simulink model "four_machine"  (R2020a)
settings: Solver=ode15s  StartTime=0.0  StopTime=20  MaxStep=1/60  RelTol=1e-3  EnableMultiTasking=on
values from neighbouring files (symbols this model uses):
  case_n = i-1    [main_simulations.m]
  d11_step = load_step_size    (= 350)    [main_simulations.m]
  d5_step = 0    [main_simulations.m]
  H = [6.5 6.5 6.175 6.175]*.75    [main_simulations.m]
  kpss = 0.2    [main_simulations.m]
  Tdelay = 0.2    [main_simulations.m]
undefined symbols (not defined in the file or in its folder): D1, d_rad, Delta, K
libraries: powerlib x49, sps_avr x4, powerlib_meascontrol x4, simulink x2, dspsigops x2
(part 1 of 2)
Description:
  | Copyright 2008-2018 The MathWorks, Inc.
settings Model: FPTRunName=Active  ExtModeTrigMode=oneshot  ExtModeArmWhenConnect=off  ExtModeAutoUpdateStatusClock=off  Creator=MathWorks  LastModifiedBy=joakbj
settings DataIOCC: SaveFormat=Array  SaveOutput=off  SaveTime=off  ReturnWorkspaceOutputs=off  TimeSaveName=t  SignalLoggingName=sigsOut
settings OptimizationCC: BlockReduction=off  BooleanDataType=off  ExpressionDepthLimit=2147483647  InitFltsAndDblsToZero=on  LifeSpan=inf
settings DebuggingCC: UnderspecifiedInitializationDetection=Classic  MergeDetectMultiDrivingBlocksExec=none  SignalResolutionControl=TryResolveAllWithWarning  MultiTaskDSMMsg=warning  MultiTaskCondExecSysMsg=none  FcnCallInpInsideContextMsg=warning  UnconnectedInputMsg=none  UnconnectedOutputMsg=none  UnconnectedLineMsg=none  StateNameClashWarn=warning  SFUnexpectedBacktrackingDiag=warning  SFNoUnconditionalDefaultTransitionDiag=warning  SFExecutionAtInitializationDiag=none  ArithmeticOperatorsInVariantConditions=warning
settings HardwareCC: ProdBitPerPointer=32  ProdBitPerSizeT=32  ProdBitPerPtrDiffT=32  ProdLargestAtomicFloat=None  ProdIntDivRoundTo=Undefined  ProdEndianess=Unspecified  ProdWordSize=32  ProdHWDeviceType=32-bit Generic  TargetUnknown=on
settings ModelReferenceCC: PropagateSignalLabelsOutOfModel=off
settings SFSimCC: SimUseLocalCustomCode=off  CustomCodeUndefinedFunction=UseInterfaceOnly
settings RTWCC: RTWUseLocalCustomCode=off
settings CodeAppCC: StateflowObjectComments=on
settings GRTTargetCC: TargetLangStandard=C89/C90 (ANSI)  CombineOutputUpdateFcns=off  GRTInterface=on
settings ConfigComp: CovMetricSettings=dw  CovHtmlReporting=on  CovSaveCumulativeToWorkspaceVar=on  CovSaveSingleToWorkspaceVar=on  CovExternalEMLEnable=off  CovSFcnEnable=off
settings SimscapeCC: SimscapeNormalizeSystem=off

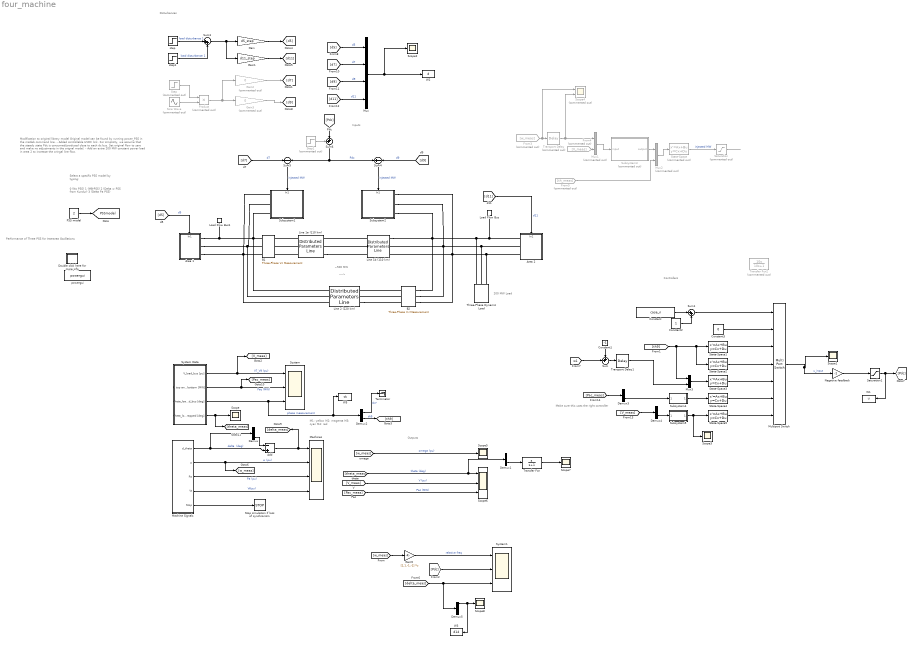
== system four_machine ==
  note: Modification to original library model
      | Original model can be found by running power_PSS in the matlab command line.
      |
      | - Added controllable HVDC link. For simplisity, we assume that the steady state Pdc is
      | consumed/produced close to each dc bus.
      | Set original flow to zero and make no adjustments in the orignal model.
      |
      | - Add an extra 200 MW constant power load in area 2 to increase the oringal line flow.
  note: Make sure this uses the right controller
  note: 200 MW Load
  note: Disturbances
  note: Performance of Three PSS for Interarea Oscillations
  note: M1: yellow
      | M2: magenta
      | M3: cyan
      | M4: red
  note: ---->
  note: ~500 MW
  note: Select a specific PSS model
      | by typing:
  note: 0  (No PSS)
      | 1  (MB-PSS)
      | 2  (Delta w PSS from Kundur)
      | 3  (Delta Pa PSS)
  note: Outputs
  note: Inputs
  note: Controllers
  Add : Sum  Inputs=-+
  Area 1 : Subsystem
      settings: PortSchema="{\"entries\":[{\"content\":{\"sides\":[{\"content\":{\"connectorIds\":[]},\"type\":\"ConnectorPlacement.EquallySpacedRectSide\",\"uuid\":\"61530743-916b-41d3-ae4c-b0f59ade86dc\"},{\"content\":{\"connectorIds\":[\"RConn1\",\"RConn2\",\"RConn3\"],\"side\":\"RIGHT\"},\"type\":\"ConnectorPlacement.EquallySpacedRectSide\",\"uuid\":\"d4cdbb0d-3031-41c4-8349-05093edd83c9\"},{\"content\":{\"connectorIds\":[\"In1\"],\"side\":\"TOP\"},\"type\":\"ConnectorPlacement.EquallySpacedRectSide\",\"uuid\":\"5f7b4922-b9b9-47cc-81cb-58a7e8a20879\"}]},\"type\":\"ConnectorPlacement.EquallySpacedConnector\",\"uuid\":\"5acf2a3c-d6e4-438f-a169-9a860cbc2f6d\"}],\"packageUris\":[\"http://schema.mathworks.com/mf0/Connector/19700101\"],\"version\":\"1.0\"}"
  Area 2 : Subsystem
      settings: PortSchema="{\"entries\":[{\"content\":{\"sides\":[{\"content\":{\"connectorIds\":[\"LConn1\",\"LConn2\",\"LConn3\"]},\"type\":\"ConnectorPlacement.EquallySpacedRectSide\",\"uuid\":\"e7faa0ec-56a1-4760-94c0-742828807d5f\"},{\"content\":{\"connectorIds\":[],\"side\":\"RIGHT\"},\"type\":\"ConnectorPlacement.EquallySpacedRectSide\",\"uuid\":\"ccb950ba-2df4-4215-8f92-1b8fc73c9261\"},{\"content\":{\"connectorIds\":[\"In1\"],\"side\":\"TOP\"},\"type\":\"ConnectorPlacement.EquallySpacedRectSide\",\"uuid\":\"43b0d608-fcb4-47fa-8870-be4e09a9c317\"}]},\"type\":\"ConnectorPlacement.EquallySpacedConnector\",\"uuid\":\"da59aa7b-0e3d-4680-8192-ce0c0266e238\"}],\"packageUris\":[\"http://schema.mathworks.com/mf0/Connector/19700101\"],\"version\":\"1.0\"}"
  B1 : powerlib/Measurements/Three-Phase V-I Measurement  VoltageMeasurement=phase-to-ground  SetLabelV=on  LabelV=Vabc_B1  Vpu=off  VpuLL=off  CurrentMeasurement=yes  SetLabelI=on  LabelI=Iabc_B1  Ipu=off  Pbase=100e6  Vbase=500e3  OutputType=Complex  PhasorSimulation=on  PSBequivalent=0
  B2 : powerlib/Measurements/Three-Phase V-I Measurement  VoltageMeasurement=phase-to-ground  SetLabelV=on  LabelV=Vabc_B2  Vpu=off  VpuLL=off  CurrentMeasurement=yes  SetLabelI=on  LabelI=Iabc_B2  Ipu=off  Pbase=100e6  Vbase=500e3  OutputType=Complex  PhasorSimulation=on  PSBequivalent=0
  Constant : Constant  Value=case_n
  Constant1 : Constant  Value=-1
  Constant2 : Constant
  Constant3 : Constant  Value=0
  Demux : Demux
  Demux{1..4} (4 alike) : Demux  Outputs=2
  Demux5 : Demux
  Double click here for more info : Subsystem
      settings: OpenFcn=showdemo(bdroot(gcb))
      mask Display: disp('?')
  From3 : From  Commented=on  GotoTag=w_meas
  From4 : From  Commented=on  GotoTag=V_meas
  From5 : From  Commented=on  GotoTag=th_meas
  Gain : Gain  Gain=d5_step
  Gain1 : Gain  Gain=d11_step
  Gain2 : Gain  Commented=on  Gain=0
  Gain3 : Gain  Commented=on  Gain=0
  Gain5 : Gain  Gain=[1,1,-1,-1]  Multiplication=Matrix(K*u)
  Line 1a (110 km) : powerlib/Elements/Distributed Parameters Line  Phases=3  Frequency=60  Resistance=[0.0001*529 1.61]  Inductance=[0.001*529/(377) 0.0061]  Capacitance=[0.00175/529/(377) 5.2489e-9]  Length=110  x1=[1.06729153263772e-08 221955.058861017 221954.627346652;376.991118430775 376.991118430775 376.991118430775;1.05676853901888 0.612824326191211 -0.957969932782551]  x2=[8.0985690030452e-09 213828.873062733 213828.517746943;376.991118430775 376.991118430775 376.991118430775;2.81156380356507 0.285316090081509 -1.28547863099569]  x3=[4.33186807668859e-11 672.907969274506 672.908308948858;376.991118430775 376.991118430775 376.991118430775;2.44599649138148 -2.79060184246198 1.92179081798774]  x4=[3.70403487092246e-11 1739.09783381054 1739.09622903984;376.991118430775 376.991118430775 376.991118430775;-0.503630789857306 0.368243197878753 -1.20255060629328]  x5=0.000622431770558027  V1=ones(3,3)  V2=ones(3,3)  I1=ones(3,3)  I2=ones(3,3)  nHarmo=1  Measurements=None
      settings: AttributesFormatString=\n
  Line 1b (110 km) : powerlib/Elements/Distributed Parameters Line  Phases=3  Frequency=60  Resistance=[0.0001*529 1.61]  Inductance=[0.001*529/(377) 0.0061]  Capacitance=[0.00175/529/(377) 5.2489e-9]  Length=110  x1=[8.0985690030452e-09 213828.873062733 213828.517746943;376.991118430775 376.991118430775 376.991118430775;2.81156380356507 0.285316090081509 -1.28547863099569]  x2=[2.03288713597303e-08 224486.996647561 224486.735562946;376.991118430775 376.991118430775 376.991118430775;-2.93072446072062 -0.036243603410852 -1.60703851965793]  x3=[4.90350656664839e-11 690.468793518143 690.469123207699;376.991118430775 376.991118430775 376.991118430775;2.69719045221346 -2.64610173593933 2.06629090472881]  x4=[2.93087705700001e-11 1721.59813744144 1721.59654310193;376.991118430775 376.991118430775 376.991118430775;-0.775070749600102 0.222153439297898 -1.34864036891686]  x5=0.000622431770558027  V1=ones(3,3)  V2=ones(3,3)  I1=ones(3,3)  I2=ones(3,3)  nHarmo=1  Measurements=None
      settings: AttributesFormatString=\n
  Line 2 (220 km) : powerlib/Elements/Distributed Parameters Line  Phases=3  Frequency=60  Resistance=[0.0001*529 1.61]  Inductance=[0.001*529/(377) 0.0061]  Capacitance=[0.00175/529/(377) 5.2489e-9]  Length=220  x1=[1.06729153263771e-08 221955.058861017 221954.627346652;376.991118430775 376.991118430775 376.991118430775;0.822117289689359 0.467311432234616 -1.10348282673915]  x2=[2.03288713597303e-08 224486.996647561 224486.735562946;376.991118430775 376.991118430775 376.991118430775;3.11780959712945 -0.181756497367447 -1.75255141361452]  x3=[3.92860528810386e-11 669.98397742558 669.984311456636;376.991118430775 376.991118430775 376.991118430775;2.21193561854868 -2.93582336415306 1.77656929025843]  x4=[2.78977153806267e-11 1707.24475294082 1707.24317306548;376.991118430775 376.991118430775 376.991118430775;-0.986304993466549 0.0767584445474056 -1.49403536252848]  x5=0.00124486354111605  V1=ones(3,3)  V2=ones(3,3)  I1=ones(3,3)  I2=ones(3,3)  nHarmo=1  Measurements=None
      settings: AttributesFormatString=\n
  Load Flow Bus : powerlib/Measurements/Load Flow Bus  LConnTagsString=a  Phases=single  Connectors=on one side  ID=B2  Vbase=230e3  Vref=1  Vangle=0  VLF=0.976  VLFb=1  VLFc=1  angleLF=-23.74  angleLFb=0  angleLFc=0
      settings: AttributesFormatString=%<ID>\n%<Vbase>V\n%<VLF>pu\n%<angleLF>deg.
  Load Flow Bus1 : powerlib/Measurements/Load Flow Bus  LConnTagsString=a  Phases=single  Connectors=on one side  ID=B1  Vbase=230e3  Vref=1  Vangle=0  VLF=0.965  VLFb=1  VLFc=1  angleLF=13.45  angleLFb=0  angleLFc=0
      settings: AttributesFormatString=%<ID>\n%<Vbase>V\n%<VLF>pu\n%<angleLF>deg.
  Machine Signals : Subsystem
  Machines : Scope  NumInputPorts=4
  Multiport Switch : MultiPortSwitch  Inputs=6  InputSameDT=on
  Mux : Mux
  Mux1 : Mux  Commented=on  Inputs=2
  Mux2 : Mux  Commented=on  Inputs=2
  Mux3 : Mux  Inputs=2
  Negative feedback : Gain  Gain=-1
  PSS model : Constant  Value=2
  Product : Product  Commented=on
  Saturation : Saturate  Commented=on  UpperLimit=75  LowerLimit=-75
  Saturation1 : Saturate  UpperLimit=75  LowerLimit=-75
  Scope{,1..3,5,7..8} (7 alike) : Scope
  Scope4 : Scope  Commented=on  NumInputPorts=2
  Scope6 : Scope  NumInputPorts=3
  Sine Wave : Sin  Commented=on  Frequency=d_rad  Phase=-d_rad  SampleTime=0
  State-Space : StateSpace  Commented=on  A=K.A  B=K.B  C=K.C  D=K.D  InitialCondition=0
  State-Space1 : StateSpace  A=K{1}.A  B=K{1}.B  C=K{1}.C  D=K{1}.D  InitialCondition=0
  State-Space2 : StateSpace  A=K{2}.A  B=K{2}.B  C=K{2}.C  D=K{2}.D  InitialCondition=0
  State-Space3 : StateSpace  A=K{3}.A  B=K{3}.B  C=K{3}.C  D=K{3}.D  InitialCondition=0
  State-Space4 : StateSpace  A=K{4}.A  B=K{4}.B  C=K{4}.C  D=K{4}.D  InitialCondition=0
  State-Space5 : StateSpace  A=K{5}.A  B=K{5}.B  C=K{5}.C  D=K{5}.D  InitialCondition=0
  Step : Step  Commented=on  SampleTime=0
  Step1 : Step  Commented=on  After=100  SampleTime=0
  Stop simulation if loss of synchronism : Stop
  Subsystem1 : Subsystem
      settings: PortSchema="{\"entries\":[{\"content\":{\"sides\":[{\"content\":{\"connectorIds\":[\"LConn1\",\"LConn2\",\"LConn3\"]},\"type\":\"ConnectorPlacement.EquallySpacedRectSide\",\"uuid\":\"e7faa0ec-56a1-4760-94c0-742828807d5f\"},{\"content\":{\"connectorIds\":[],\"side\":\"RIGHT\"},\"type\":\"ConnectorPlacement.EquallySpacedRectSide\",\"uuid\":\"ccb950ba-2df4-4215-8f92-1b8fc73c9261\"},{\"content\":{\"connectorIds\":[\"In1\"],\"side\":\"TOP\"},\"type\":\"ConnectorPlacement.EquallySpacedRectSide\",\"uuid\":\"43b0d608-fcb4-47fa-8870-be4e09a9c317\"}]},\"type\":\"ConnectorPlacement.EquallySpacedConnector\",\"uuid\":\"da59aa7b-0e3d-4680-8192-ce0c0266e238\"}],\"packageUris\":[\"http://schema.mathworks.com/mf0/Connector/19700101\"],\"version\":\"1.0\"}"
  Subsystem2 : Subsystem
      settings: PortSchema="{\"entries\":[{\"content\":{\"sides\":[{\"content\":{\"connectorIds\":[\"LConn1\",\"LConn2\",\"LConn3\"]},\"type\":\"ConnectorPlacement.EquallySpacedRectSide\",\"uuid\":\"e7faa0ec-56a1-4760-94c0-742828807d5f\"},{\"content\":{\"connectorIds\":[],\"side\":\"RIGHT\"},\"type\":\"ConnectorPlacement.EquallySpacedRectSide\",\"uuid\":\"ccb950ba-2df4-4215-8f92-1b8fc73c9261\"},{\"content\":{\"connectorIds\":[\"In1\"],\"side\":\"TOP\"},\"type\":\"ConnectorPlacement.EquallySpacedRectSide\",\"uuid\":\"43b0d608-fcb4-47fa-8870-be4e09a9c317\"}]},\"type\":\"ConnectorPlacement.EquallySpacedConnector\",\"uuid\":\"da59aa7b-0e3d-4680-8192-ce0c0266e238\"}],\"packageUris\":[\"http://schema.mathworks.com/mf0/Connector/19700101\"],\"version\":\"1.0\"}"
  Subsystem3 : Subsystem  Commented=on
  Subsystem4 : Subsystem
  Subsystem5 : Subsystem
  Sum : Sum  Inputs=++|
  Sum1 : Sum  Inputs=|++
  Sum3 : Sum  Inputs=|++
  Sum4 : Sum  Inputs=+|-
  Sum5 : Sum  Inputs=-|-
  Sum6 : Sum  Inputs=++|
  System : Scope  NumInputPorts=3
  System Data : Subsystem
  System1 : Scope  NumInputPorts=3
  Terminator : Terminator
  Three-Phase Dynamic Load : powerlib/Elements/Three-Phase Dynamic Load  NominalVoltage=[ 230e3 60 ]  ActiveReactivePowers=[2e+08 2.22045e-08]  PositiveSequence=[0.97603 -23.7392]  ExternalControl=off  NpNq=[0 0]  TimeConstants="[0  0  0  0]"  MinimumVoltage=0.7  Tfilter=1e-4  LoadFlowParameters=[4,0,0,0,0]
      settings: SourceProductBaseCode=PS
  Transfer Fcn : TransferFcn  Numerator=[1 0]  Denominator=[1 1]
  Transfer Fcn2 : TransferFcn  Commented=on  Numerator=[10 0]  Denominator=[10 1]
  Transport Delay : TransportDelay  Commented=on  DelayTime=Tdelay  InitialOutput=1  TransDelayFeedthrough=on
  Transport Delay1 : TransportDelay  DelayTime=Tdelay  TransDelayFeedthrough=on
  W1 : ToWorkspace  VariableName=u  SampleTime=1/60
  W2 : ToWorkspace  VariableName=d  SampleTime=1/60
  W3 : ToWorkspace  VariableName=d14  SampleTime=1/60
  W5 : ToWorkspace  VariableName=th  SampleTime=1/60
  powergui : powerlib/powergui  Priority=2  SimulationMode=Phasor  SampleTime=0  frequency=60  Iterations=50  frequencyindice=60  Pbase=100e6  ErrMax=0.0001  UnitsV=kV  UnitsW=MW  buscounter=0  FunctionMessages=off  echomessages=off  EnableUseOfTLC=off  CurrentSourceSwitches=off  DisableSnubberDevices=off  DisableRonSwitches=off  DisableVfSwitches=off  DisplayEquations=off  AutomaticDiscreteSolvers=off  SolverType=Tustin  Interpol=off  ExternalGateDelay=off  methode=off  Ts=0  x0status=blocks  SPID=off  SwTol=0  HookPort=off  NonlinearTolerance=1e-4  nMaxIteration=100  ContinueOnMaxIteration=off  RestoreLinks=warning  ResistiveCurrentMeasurement=off  Frange=logspace(0,3,50)  Ylog=off  Xlog=off  ShowGrid=off  save=off  variable=ZData  structure=0  ZoomFFT=on  StartTime=0.0  cycles=1  DisplayStyle=1  fundamental=60  FreqAxis=off  MaxFrequency=1000  frequencyindicesteady=1  RmsSteady=1  display=off
  step : Step  SampleTime=0
  step1 : Step  Time=2  After=-1  SampleTime=0
  tag scope: PSSmodel=global
  wires:
  Machine Signals/1(d_theta) -> Add/2, Demux/1  "delta  (deg)"
  Machine Signals/2(w) -> [w_meas], Machines/2  "w (pu)"
  Machine Signals/3(Pa) -> Machines/3  "Pa (pu)"
  Machine Signals/4(Vt) -> Machines/4  "Vt(pu)"
  Machine Signals/5(Stop) -> Stop simulation if loss of synchronism/1
  System Data/1(V_load_bus [pu]) -> [V_meas], System/1  "V7_V9 (pu)"
  System Data/2(P top and bottom [MW]) -> [Pac_meas], System/2  "Pac (MW)"
  PSS model/1 -> [PSSmodel]
  [d11] -> Area 2/1(In1)  "d11"
  Sum4/1 -> Subsystem2/1(In1)  "injected MW"
  [d5] -> Area 1/1(In1)  "d5"
  Sum5/1 -> Subsystem1/1(In1)  "injected MW"
  System Data/4(theta_load_bus wrapped [deg]) -> [theta_meas], Scope/1
  Sine Wave/1 -> Product/2
  Step/1 -> Product/1
  Product/1 -> Gain2/1, Gain3/1
  System Data/3(theta_load_bus [deg]) -> Demux2/1, W5/1, System/3  "phase measurement"
  step/1 -> Sum3/1  "load disturbance 1"
  step1/1 -> Sum3/2  "load disturbance 1"
  Sum3/1 -> Gain1/1, Gain/1
  Gain5/1 -> System1/1  "relative freq"
  From3/1 -> Scope4/1, Transport Delay/1
  From4/1 -> Mux1/2
  From5/1 -> Mux2/2
  Mux1/1 -> Subsystem3/1(input)
  State-Space/1 -> Saturation/1  "injected MW"
  Mux/1 -> W2/1, Scope2/1
  Subsystem3/1(output) -> Mux2/1
  Mux2/1 -> State-Space/1
  Transport Delay/1 -> Scope4/2, Mux1/1
  Saturation/1 -> ?
  [d7] -> Sum5/1  "d7"
  [d9] -> Sum4/2  "d9"
  Gain2/1 -> [d7]
  [w_meas] -> Gain5/1
  Demux/4 -> Add/1
  Add/1 -> Machines/1, [delta_meas]
  [Pdc] -> Sum6/2
  Step1/1 -> Sum6/1
  Sum6/1 -> Sum5/2, Sum4/1  "Pdc"
  Gain/1 -> [d5]
  Gain1/1 -> [d11]
  [d5] -> Mux/1  "d5"
  [d7] -> Mux/2  "d7"
  [d9] -> Mux/3  "d9"
  [d11] -> Mux/4  "d11"
  [w_meas] -> Scope5/1  "omega (pu)"
  [theta_meas] -> Demux1/1, Scope6/1  "theta (deg)"
  [V_meas] -> Scope6/2  "V (pu)"
  [Pac_meas] -> Scope6/3  "Pac (MW)"
  Gain3/1 -> [d9]
  Transfer Fcn/1 -> Scope7/1
  Demux1/2 -> Transfer Fcn/1
  Multiport Switch/1 -> Negative feedback/1, Scope1/1  "u_input"
  Demux2/2 -> [th9]  "th9"
  [th9] -> State-Space2/1, State-Space1/1, Mux3/1
  [Pdc] -> System1/2
  Negative feedback/1 -> Saturation1/1
  Saturation1/1 -> W1/1, [Pdc]
  Mux3/1 -> State-Space3/1
  [w1] -> Sum/2
  Sum/1 -> Transport Delay1/1
  Transport Delay1/1 -> Mux3/2
  [Pac_meas] -> Demux3/1
  [V_meas] -> Demux4/1
  Constant1/1 -> Sum/1
  Subsystem4/1(output) -> State-Space4/1
  Demux4/2 -> Subsystem5/1(input)
  Subsystem5/1(output) -> Scope3/1, State-Space5/1
  Demux3/2 -> Subsystem4/1(input)
  [delta_meas] -> Demux5/1, System1/3
  Demux5/1 -> W3/1, Scope8/1
  State-Space5/1 -> Multiport Switch/7
  State-Space4/1 -> Multiport Switch/6
  State-Space3/1 -> Multiport Switch/5
  State-Space2/1 -> Multiport Switch/4
  State-Space1/1 -> Multiport Switch/3
  Constant/1 -> Sum1/1
  Sum1/1 -> Multiport Switch/1
  Constant2/1 -> Sum1/2
  Constant3/1 -> Multiport Switch/2
  Demux2/1 -> Terminator/1  "th7"
  connections:
  Line 1b (110 km)/LConn1 -- Line 1a (110 km)/RConn1
  Line 1b (110 km)/LConn2 -- Line 1a (110 km)/RConn2
  Line 1a (110 km)/RConn3 -- Line 1b (110 km)/LConn3
  Three-Phase Dynamic Load/LConn2 -- Subsystem2/LConn2 -- B2/RConn2 -- Line 1b (110 km)/RConn2 -- Area 2/LConn2
  Three-Phase Dynamic Load/LConn1 -- Area 2/LConn1 -- Load Flow Bus/LConn1 -- Subsystem2/LConn3 -- B2/RConn1 -- Line 1b (110 km)/RConn1
  Three-Phase Dynamic Load/LConn3 -- Subsystem2/LConn1 -- Line 1b (110 km)/RConn3 -- B2/RConn3 -- Area 2/LConn3
  B2/LConn1 -- Line 2 (220 km)/RConn1
  B2/LConn2 -- Line 2 (220 km)/RConn2
  Line 2 (220 km)/RConn3 -- B2/LConn3
  Area 1/RConn1 -- B1/LConn1 -- Line 2 (220 km)/LConn1 -- Subsystem1/LConn3 -- Load Flow Bus1/LConn1
  Area 1/RConn2 -- B1/LConn2 -- Subsystem1/LConn2 -- Line 2 (220 km)/LConn2
  Area 1/RConn3 -- B1/LConn3 -- Line 2 (220 km)/LConn3 -- Subsystem1/LConn1
  Line 1a (110 km)/LConn1 -- B1/RConn1
  Line 1a (110 km)/LConn2 -- B1/RConn2
  Line 1a (110 km)/LConn3 -- B1/RConn3

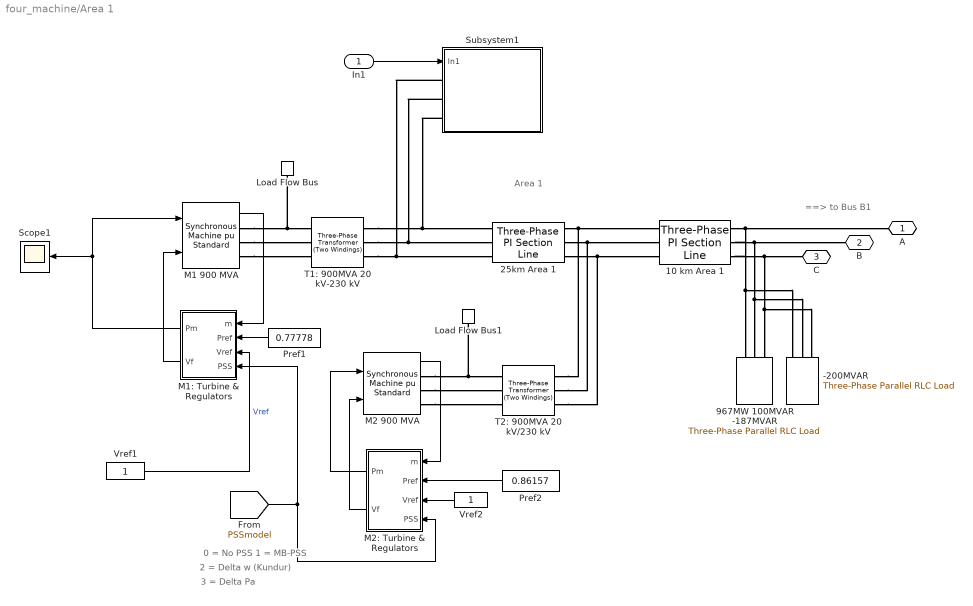
== system four_machine/Area 1 ==
  note: Area 1
  note: ==> to Bus B1
  note: 0 = No PSS
      | 1 = MB-PSS
  note: 3 = Delta Pa
  note: 2 = Delta w (Kundur)
  In1 : Inport
  -200MVAR : powerlib/Elements/Three-Phase Parallel RLC Load  LConnTagsString=A|B|C  Configuration=Y (grounded)  NominalVoltage=230e3  Vabc=[1e3 1e3 1e3]  Vabcp=[1e3 1e3 1e3]  NominalFrequency=60  UnbalancedPower=off  ActivePower=0  InductivePower=0  CapacitivePower=200e6  Pabc=[10e3 9e3 11e3]  QLabc=[100 90 110]  QCabc=[100 90 110]  Pabcp=[10e3 9e3 11e3]  QLabcp=[100 90 110]  QCabcp=[100 90 110]  Measurements=None  LoadType=constant Z
  10 km Area 1 : powerlib/Elements/Three-Phase PI Section Line  LConnTagsString=a|b|c  RConnTagsString=A|B|C  Frequency=60  Resistances=[0.0001*529 1.61]  Inductances=[0.001*529/(377) 0.0061]  Capacitances=[0.00175/529/(377) 5.2489e-9]  Length=10
  25km Area 1 : powerlib/Elements/Three-Phase PI Section Line  LConnTagsString=a|b|c  RConnTagsString=A|B|C  Frequency=60  Resistances=[0.0001*529 1.61]  Inductances=[0.001*529/(377) 0.0061]  Capacitances=[0.00175/529/(377) 5.2489e-9]  Length=25
  967MW 100MVAR -187MVAR : powerlib/Elements/Three-Phase Parallel RLC Load  LConnTagsString=A|B|C  Configuration=Y (grounded)  NominalVoltage=230e3  Vabc=[1e3 1e3 1e3]  Vabcp=[1e3 1e3 1e3]  NominalFrequency=60  UnbalancedPower=off  ActivePower=967000000  InductivePower=100e6  CapacitivePower=187e6  Pabc=[10e3 9e3 11e3]  QLabc=[100 90 110]  QCabc=[100 90 110]  Pabcp=[10e3 9e3 11e3]  QLabcp=[100 90 110]  QCabcp=[100 90 110]  Measurements=None  LoadType=constant Z
  Load Flow Bus : powerlib/Measurements/Load Flow Bus  LConnTagsString=a  Phases=single  Connectors=on one side  ID=M1_Area1  Vbase=20e3  Vref=1  Vangle=0  VLF=1  VLFb=1  VLFc=1  angleLF=9.585  angleLFb=0  angleLFc=0
      settings: AttributesFormatString=%<ID>\n%<Vbase>V\n%<VLF>pu\n%<angleLF>deg.
  Load Flow Bus1 : powerlib/Measurements/Load Flow Bus  LConnTagsString=a  Phases=single  Connectors=on one side  ID=M2_Area1  Vbase=20e3  Vref=1  Vangle=0  VLF=1  VLFb=1  VLFc=1  angleLF=0  angleLFb=0  angleLFc=0
      settings: AttributesFormatString=%<ID>\n%<Vbase>V\n%<VLF>pu\n%<angleLF>deg.
  M1 900 MVA : powerlib/Machines/Synchronous Machine pu Standard  PresetModel=No  MechanicalLoad=Mechanical power Pm  ShowDetailedParameters=on  RotorType=Round  Units=per unit standard parameters  MeasurementBus=off  NominalParameters="[900E6  20000   60 ]"  Reactances1=[1.8 .3 .25 1.7 .55 .25 .2]  Reactances2=[ 1.305, 0.296, 0.252, 0.474, 0.243, 0.18 ]  dAxisTimeConstants=Open-circuit  qAxisTimeConstants=Open-circuit  TimeConstants1=[]  TimeConstants2=[8 .03 .4 .05]  TimeConstants3=[]  TimeConstants4=[]  TimeConstants5=[ 1.01, 0.053, 0.1 ]  TimeConstants6=[]  TimeConstants7=[]  TimeConstants8=[]  StatorResistance=0.0025  Mechanical=[ H(1) 0 4]  PolePairs=4  InitialConditions=[0 -33.7715 0.791144 0.791144 0.791144 -0.961842 -120.962 119.038 1.88449]  SetSaturation=off  Saturation=[0.6404,0.7127,0.8441,0.9214,0.9956,1.082,1.19,1.316,1.457;0.7,0.7698,0.8872,0.9466,0.9969,1.046,1.1,1.151,1.201]  LoadFlowParameters=[1 700000000 0 0 0]  TsPowergui=0  TsBlock=-1  IterativeModel=Trapezoidal non iterative  IterativeDiscreteModel=Trapezoidal non iterative  BusType=PV  Pref=700000000  Qref=0  Qmin=-Inf  Qmax=Inf  PLF=0  QLF=0
      settings: AttributesFormatString=\n\n
  M1: Turbine & Regulators : Subsystem
  M2 900 MVA : powerlib/Machines/Synchronous Machine pu Standard  PresetModel=No  MechanicalLoad=Mechanical power Pm  ShowDetailedParameters=on  RotorType=Round  Units=per unit standard parameters  MeasurementBus=off  NominalParameters="[900E6  20000   60 ]"  Reactances1=[1.8 .3 .25 1.7 .55 .25 .2]  Reactances2=[ 1.305, 0.296, 0.252, 0.474, 0.243, 0.18 ]  dAxisTimeConstants=Open-circuit  qAxisTimeConstants=Open-circuit  TimeConstants1=[]  TimeConstants2=[8 .03 .4 .05]  TimeConstants3=[]  TimeConstants4=[]  TimeConstants5=[ 1.01, 0.053, 0.1 ]  TimeConstants6=[]  TimeConstants7=[]  TimeConstants8=[]  StatorResistance=0.0025  Mechanical=[ H(2) 0 4]  PolePairs=4  InitialConditions=[0 -44.1333 0.896015 0.896015 0.896015 -15.9379 -135.938 104.062 2.11884]  SetSaturation=off  Saturation=[0.6404,0.7127,0.8441,0.9214,0.9956,1.082,1.19,1.316,1.457;0.7,0.7698,0.8872,0.9466,0.9969,1.046,1.1,1.151,1.201]  LoadFlowParameters=[2 700000000 0 0 0]  TsPowergui=0  TsBlock=-1  IterativeModel=Trapezoidal non iterative  IterativeDiscreteModel=Trapezoidal non iterative  BusType=swing  Pref=0  Qref=0  Qmin=-Inf  Qmax=Inf  PLF=0  QLF=0
      settings: AttributesFormatString=\n\n
  M2: Turbine & Regulators : Subsystem
  Pref1 : Constant  Value=0.77778
  Pref2 : Constant  Value=0.86157
  Scope1 : Scope
  Subsystem1 : Subsystem
  T1: 900MVA 20 kV-230 kV : powerlib/Elements/Three-Phase Transformer (Two Windings)  Winding1Connection=Delta (D1)  Winding2Connection=Yg  CoreType=Three single-phase transformers  SetSaturation=off  Hysteresis=off  DataFile='hysteresis'  SetInitialFlux=off  Measurements=None  UNITS=pu  NominalPower="[ 900e6   60 ]"  Winding1="[ 20e3  1e-6   0  ]"  Winding2="[ 230e3  1e-6   0.15 ]"  Rm=500  Lm=500  L0=0.5  Saturation="[ 0,0  ;  0.005,1.2  ;  1.0,1.4 ]"  InitialFluxes=[ 0.8 , -0.8 , 0.7 ]  BreakLoop=off  DiscreteSolver=Trapezoidal iterative  DataType=off  TransfoNumber=0
  T2: 900MVA 20 kV/230 kV : powerlib/Elements/Three-Phase Transformer (Two Windings)  Winding1Connection=Delta (D1)  Winding2Connection=Yg  CoreType=Three single-phase transformers  SetSaturation=off  Hysteresis=off  DataFile='hysteresis'  SetInitialFlux=off  Measurements=None  UNITS=pu  NominalPower=[ 900e6 60 ]  Winding1="[ 20e3 1e-6  0.0]"  Winding2=[ 230e3 1e-6 0.15]  Rm=500  Lm=500  L0=0.5  Saturation="[ 0,0  ;  0.005,1.2  ;  1.0,1.4 ]"  InitialFluxes=[ 0.8 , -0.8 , 0.7 ]  BreakLoop=off  DiscreteSolver=Trapezoidal iterative  DataType=off  TransfoNumber=0
  Vref1 : Constant
  Vref2 : Constant
  " A" : PMIOPort  Side=Right
  " B" : PMIOPort  Port=2  Side=Right
  " C" : PMIOPort  Port=3  Side=Right
  wires:
  Pref1/1 -> M1: Turbine & Regulators/2(Pref)
  Vref1/1 -> M1: Turbine & Regulators/3(Vref)  "Vref"
  [PSSmodel] -> M1: Turbine & Regulators/4(PSS), M2: Turbine & Regulators/4(PSS)
  Pref2/1 -> M2: Turbine & Regulators/2(Pref)
  Vref2/1 -> M2: Turbine & Regulators/3(Vref)
  M2 900 MVA/1 -> M2: Turbine & Regulators/1(m)
  M2: Turbine & Regulators/1(Pm) -> M2 900 MVA/1
  M2: Turbine & Regulators/2(Vf) -> M2 900 MVA/2
  M1: Turbine & Regulators/2(Vf) -> M1 900 MVA/2
  M1 900 MVA/1 -> M1: Turbine & Regulators/1(m)
  M1: Turbine & Regulators/1(Pm) -> Scope1/1, M1 900 MVA/1
  In1/1 -> Subsystem1/1(In1)
  connections:
  T1: 900MVA 20 kV-230 kV/RConn1 -- Subsystem1/LConn3 -- 25km Area 1/LConn1
  T1: 900MVA 20 kV-230 kV/RConn2 -- Subsystem1/LConn2 -- 25km Area 1/LConn2
  M2 900 MVA/RConn1 -- T2: 900MVA 20 kV/230 kV/LConn1 -- Load Flow Bus1/LConn1
  M2 900 MVA/RConn2 -- T2: 900MVA 20 kV/230 kV/LConn2
  M2 900 MVA/RConn3 -- T2: 900MVA 20 kV/230 kV/LConn3
  T1: 900MVA 20 kV-230 kV/RConn3 -- Subsystem1/LConn1 -- 25km Area 1/LConn3
  10 km Area 1/RConn1 -- " A"/RConn1 -- 967MW 100MVAR -187MVAR/LConn1 -- -200MVAR/LConn1
  10 km Area 1/RConn2 -- " B"/RConn1 -- 967MW 100MVAR -187MVAR/LConn2 -- -200MVAR/LConn2
  10 km Area 1/RConn3 -- " C"/RConn1 -- 967MW 100MVAR -187MVAR/LConn3 -- -200MVAR/LConn3
  M1 900 MVA/RConn1 -- T1: 900MVA 20 kV-230 kV/LConn1 -- Load Flow Bus/LConn1
  M1 900 MVA/RConn2 -- T1: 900MVA 20 kV-230 kV/LConn2
  M1 900 MVA/RConn3 -- T1: 900MVA 20 kV-230 kV/LConn3
  25km Area 1/RConn2 -- 10 km Area 1/LConn2 -- T2: 900MVA 20 kV/230 kV/RConn2
  25km Area 1/RConn1 -- 10 km Area 1/LConn1 -- T2: 900MVA 20 kV/230 kV/RConn1
  25km Area 1/RConn3 -- 10 km Area 1/LConn3 -- T2: 900MVA 20 kV/230 kV/RConn3

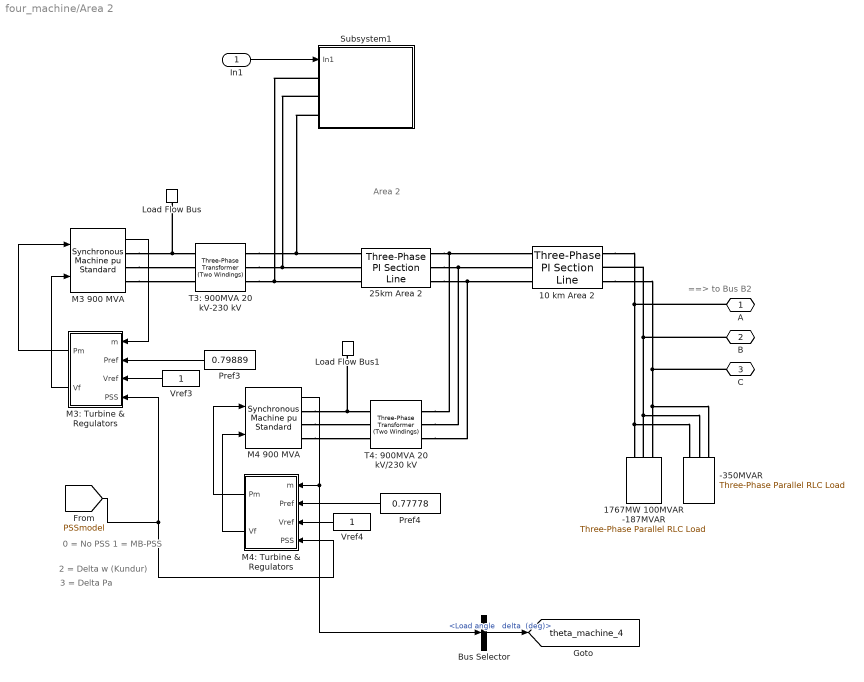
== system four_machine/Area 2 ==
  note: 2 = Delta w (Kundur)
  note: 3 = Delta Pa
  note: 0 = No PSS
      | 1 = MB-PSS
  note: ==> to Bus B2
  note: Area 2
  In1 : Inport
  -350MVAR : powerlib/Elements/Three-Phase Parallel RLC Load  LConnTagsString=A|B|C  Configuration=Y (grounded)  NominalVoltage=230e3  Vabc=[1e3 1e3 1e3]  Vabcp=[1e3 1e3 1e3]  NominalFrequency=60  UnbalancedPower=off  ActivePower=0  InductivePower=0  CapacitivePower=350e6  Pabc=[10e3 9e3 11e3]  QLabc=[100 90 110]  QCabc=[100 90 110]  Pabcp=[10e3 9e3 11e3]  QLabcp=[100 90 110]  QCabcp=[100 90 110]  Measurements=None  LoadType=constant Z
  10 km Area 2 : powerlib/Elements/Three-Phase PI Section Line  LConnTagsString=a|b|c  RConnTagsString=A|B|C  Frequency=60  Resistances=[0.0001*529 1.61]  Inductances=[0.001*529/(377) 0.0061]  Capacitances=[0.00175/529/(377) 5.2489e-9]  Length=10
  1767MW 100MVAR -187MVAR : powerlib/Elements/Three-Phase Parallel RLC Load  LConnTagsString=A|B|C  Configuration=Y (grounded)  NominalVoltage=230e3  Vabc=[1e3 1e3 1e3]  Vabcp=[1e3 1e3 1e3]  NominalFrequency=60  UnbalancedPower=off  ActivePower=1767000000  InductivePower=100e6  CapacitivePower=187e6  Pabc=[10e3 9e3 11e3]  QLabc=[100 90 110]  QCabc=[100 90 110]  Pabcp=[10e3 9e3 11e3]  QLabcp=[100 90 110]  QCabcp=[100 90 110]  Measurements=None  LoadType=constant Z
  25km Area 2 : powerlib/Elements/Three-Phase PI Section Line  LConnTagsString=a|b|c  RConnTagsString=A|B|C  Frequency=60  Resistances=[0.0001*529 1.61]  Inductances=[0.001*529/(377) 0.0061]  Capacitances=[0.00175/529/(377) 5.2489e-9]  Length=25
  Bus Selector : BusSelector  OutputSignals="Load angle   delta  (deg)"
  Load Flow Bus : powerlib/Measurements/Load Flow Bus  LConnTagsString=a  Phases=single  Connectors=on one side  ID=M3_Area2  Vbase=20e3  Vref=1  Vangle=0  VLF=1  VLFb=1  VLFc=1  angleLF=-27.7  angleLFb=0  angleLFc=0
      settings: AttributesFormatString=%<ID>\n%<Vbase>V\n%<VLF>pu\n%<angleLF>deg.
  Load Flow Bus1 : powerlib/Measurements/Load Flow Bus  LConnTagsString=a  Phases=single  Connectors=on one side  ID=M4_Area2  Vbase=20e3  Vref=1  Vangle=0  VLF=1  VLFb=1  VLFc=1  angleLF=-38.46  angleLFb=0  angleLFc=0
      settings: AttributesFormatString=%<ID>\n%<Vbase>V\n%<VLF>pu\n%<angleLF>deg.
  M3 900 MVA : powerlib/Machines/Synchronous Machine pu Standard  PresetModel=No  MechanicalLoad=Mechanical power Pm  ShowDetailedParameters=on  RotorType=Round  Units=per unit standard parameters  MeasurementBus=off  NominalParameters="[900E6  20000   60 ]"  Reactances1=[1.8 .3 .25 1.7 .55 .25 .2]  Reactances2=[ 1.305, 0.296, 0.252, 0.474, 0.243, 0.18 ]  dAxisTimeConstants=Open-circuit  qAxisTimeConstants=Open-circuit  TimeConstants1=[]  TimeConstants2=[8 .03 .4 .05]  TimeConstants3=[]  TimeConstants4=[]  TimeConstants5=[ 1.01, 0.053, 0.1 ]  TimeConstants6=[]  TimeConstants7=[]  TimeConstants8=[]  StatorResistance=0.0025  Mechanical=[ H(3) 0 4]  PolePairs=4  InitialConditions=[0 -69.7974 0.809772 0.809772 0.809772 -37.0997 -157.1 82.9003 1.89816]  SetSaturation=off  Saturation=[0.6404,0.7127,0.8441,0.9214,0.9956,1.082,1.19,1.316,1.457;0.7,0.7698,0.8872,0.9466,0.9969,1.046,1.1,1.151,1.201]  LoadFlowParameters=[1 719000000 0 0 0]  TsPowergui=0  TsBlock=-1  IterativeModel=Trapezoidal non iterative  IterativeDiscreteModel=Trapezoidal non iterative  BusType=PV  Pref=719000000  Qref=0  Qmin=-Inf  Qmax=Inf  PLF=0  QLF=0
      settings: AttributesFormatString=\n\n
  M3: Turbine & Regulators : Subsystem
  M4 900 MVA : powerlib/Machines/Synchronous Machine pu Standard  PresetModel=No  MechanicalLoad=Mechanical power Pm  ShowDetailedParameters=on  RotorType=Round  Units=per unit standard parameters  MeasurementBus=off  NominalParameters="[900E6  20000   60 ]"  Reactances1=[1.8 .3 .25 1.7 .55 .25 .2]  Reactances2=[ 1.305, 0.296, 0.252, 0.474, 0.243, 0.18 ]  dAxisTimeConstants=Open-circuit  qAxisTimeConstants=Open-circuit  TimeConstants1=[]  TimeConstants2=[8 .03 .4 .05]  TimeConstants3=[]  TimeConstants4=[]  TimeConstants5=[ 1.01, 0.053, 0.1 ]  TimeConstants6=[]  TimeConstants7=[]  TimeConstants8=[]  StatorResistance=0.0025  Mechanical=[ H(4) 0 4]  PolePairs=4  InitialConditions=[0 -83.5997 0.801116 0.801116 0.801116 -52.3222 -172.322 67.6778 1.94232]  SetSaturation=off  Saturation=[0.6404,0.7127,0.8441,0.9214,0.9956,1.082,1.19,1.316,1.457;0.7,0.7698,0.8872,0.9466,0.9969,1.046,1.1,1.151,1.201]  LoadFlowParameters=[1 700000000 0 0 0]  TsPowergui=0  TsBlock=-1  IterativeModel=Trapezoidal non iterative  IterativeDiscreteModel=Trapezoidal non iterative  BusType=PV  Pref=700000000  Qref=0  Qmin=-Inf  Qmax=Inf  PLF=0  QLF=0
      settings: AttributesFormatString=\n\n
  M4: Turbine & Regulators : Subsystem
  Pref3 : Constant  Value=0.79889
  Pref4 : Constant  Value=0.77778
  Subsystem1 : Subsystem
  T3: 900MVA 20 kV-230 kV : powerlib/Elements/Three-Phase Transformer (Two Windings)  Winding1Connection=Delta (D1)  Winding2Connection=Yg  CoreType=Three single-phase transformers  SetSaturation=off  Hysteresis=off  DataFile='hysteresis'  SetInitialFlux=off  Measurements=None  UNITS=pu  NominalPower="[ 900e6   60 ]"  Winding1="[ 20e3  1e-6   0  ]"  Winding2="[ 230e3  1e-6   0.15 ]"  Rm=500  Lm=500  L0=0.5  Saturation="[ 0,0  ;  0.005,1.2  ;  1.0,1.4 ]"  InitialFluxes=[ 0.8 , -0.8 , 0.7 ]  BreakLoop=off  DiscreteSolver=Trapezoidal iterative  DataType=off  TransfoNumber=0
  T4: 900MVA 20 kV/230 kV : powerlib/Elements/Three-Phase Transformer (Two Windings)  Winding1Connection=Delta (D1)  Winding2Connection=Yg  CoreType=Three single-phase transformers  SetSaturation=off  Hysteresis=off  DataFile='hysteresis'  SetInitialFlux=off  Measurements=None  UNITS=pu  NominalPower=[ 900e6 60 ]  Winding1="[ 20e3 1e-6  0.0]"  Winding2=[ 230e3 1e-6 0.15]  Rm=500  Lm=500  L0=0.5  Saturation="[ 0,0  ;  0.005,1.2  ;  1.0,1.4 ]"  InitialFluxes=[ 0.8 , -0.8 , 0.7 ]  BreakLoop=off  DiscreteSolver=Trapezoidal iterative  DataType=off  TransfoNumber=0
  Vref3 : Constant
  Vref4 : Constant
  A : PMIOPort  Side=Left
  B : PMIOPort  Port=2  Side=Left
  C : PMIOPort  Port=3  Side=Left
  tag scope: theta_machine_4=global
  wires:
  [PSSmodel] -> M3: Turbine & Regulators/4(PSS), M4: Turbine & Regulators/4(PSS)
  Pref3/1 -> M3: Turbine & Regulators/2(Pref)
  Vref3/1 -> M3: Turbine & Regulators/3(Vref)
  Pref4/1 -> M4: Turbine & Regulators/2(Pref)
  Vref4/1 -> M4: Turbine & Regulators/3(Vref)
  M3 900 MVA/1 -> M3: Turbine & Regulators/1(m)
  M3: Turbine & Regulators/2(Vf) -> M3 900 MVA/2
  M4: Turbine & Regulators/1(Pm) -> M4 900 MVA/1
  M4: Turbine & Regulators/2(Vf) -> M4 900 MVA/2
  M4 900 MVA/1 -> Bus Selector/1, M4: Turbine & Regulators/1(m)
  Bus Selector/1 -> [theta_machine_4]  "<Load angle   delta  (deg)>"
  M3: Turbine & Regulators/1(Pm) -> M3 900 MVA/1
  In1/1 -> Subsystem1/1(In1)
  connections:
  M3 900 MVA/RConn3 -- T3: 900MVA 20 kV-230 kV/LConn3
  M3 900 MVA/RConn2 -- T3: 900MVA 20 kV-230 kV/LConn2
  M3 900 MVA/RConn1 -- T3: 900MVA 20 kV-230 kV/LConn1 -- Load Flow Bus/LConn1
  T3: 900MVA 20 kV-230 kV/RConn3 -- Subsystem1/LConn1 -- 25km Area 2/LConn3
  M4 900 MVA/RConn3 -- T4: 900MVA 20 kV/230 kV/LConn3
  M4 900 MVA/RConn2 -- T4: 900MVA 20 kV/230 kV/LConn2
  M4 900 MVA/RConn1 -- T4: 900MVA 20 kV/230 kV/LConn1 -- Load Flow Bus1/LConn1
  T3: 900MVA 20 kV-230 kV/RConn2 -- Subsystem1/LConn2 -- 25km Area 2/LConn2
  T3: 900MVA 20 kV-230 kV/RConn1 -- Subsystem1/LConn3 -- 25km Area 2/LConn1
  25km Area 2/RConn2 -- 10 km Area 2/LConn2 -- T4: 900MVA 20 kV/230 kV/RConn2
  25km Area 2/RConn1 -- 10 km Area 2/LConn1 -- T4: 900MVA 20 kV/230 kV/RConn1
  25km Area 2/RConn3 -- 10 km Area 2/LConn3 -- T4: 900MVA 20 kV/230 kV/RConn3
  10 km Area 2/RConn1 -- 1767MW 100MVAR -187MVAR/LConn1 -- -350MVAR/LConn1 -- A/RConn1
  1767MW 100MVAR -187MVAR/LConn2 -- -350MVAR/LConn2 -- 10 km Area 2/RConn2 -- B/RConn1
  10 km Area 2/RConn3 -- -350MVAR/LConn3 -- 1767MW 100MVAR -187MVAR/LConn3 -- C/RConn1

== system four_machine/Double click here for more info ==

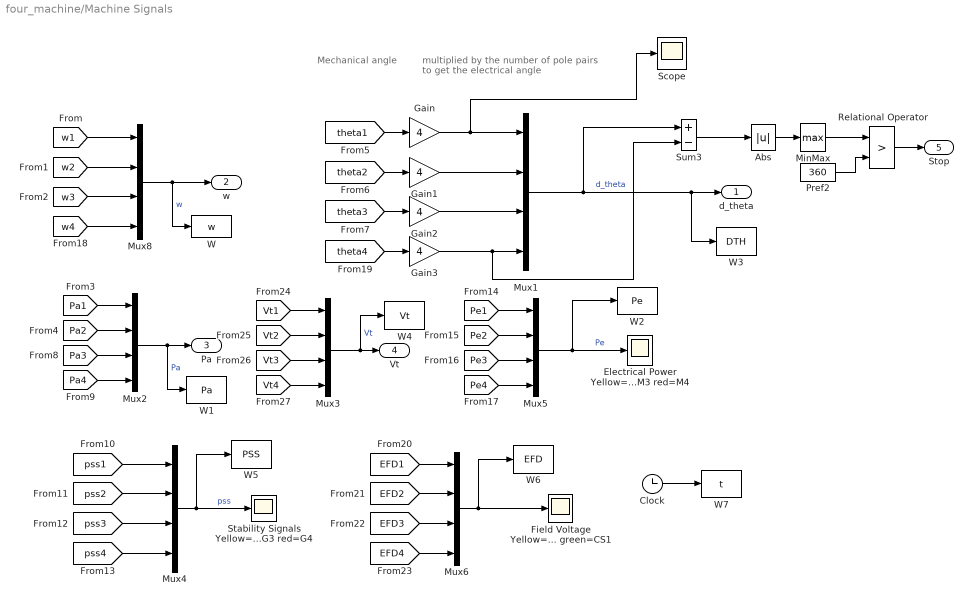
== system four_machine/Machine Signals ==
  note: Mechanical angle
  note: multiplied by the number of pole pairs
      | to get the electrical angle
  Abs : Abs  SaturateOnIntegerOverflow=on
  Clock : Clock
  "Electrical Power Yellow=M1 mag=M2 cyan=M3 red=M4 " : Scope
  Field Voltage Yellow=G1 mag=G2 cyan=G3 red=G4 green=CS1 : Scope
  Gain{,1..3} (4 alike) : Gain  Gain=4
  MinMax : MinMax  Function=max  InputSameDT=on  SaturateOnIntegerOverflow=on
  Mux{1..6,8} (7 alike) : Mux
  Pref2 : Constant  Value=360
  Relational Operator : RelationalOperator  Operator=>  RndMeth=Nearest  InputSameDT=on
  Scope : Scope
  "Stability Signals Yellow=G1 mag=G2 cyan=G3 red=G4 " : Scope
  Sum3 : Sum  Inputs=+-  InputSameDT=on  SaturateOnIntegerOverflow=on  OutDataTypeStr=Inherit: Same as first input
  W : ToWorkspace  VariableName=w  SampleTime=1/60
  W1 : ToWorkspace  VariableName=Pa  SampleTime=1/60
  W2 : ToWorkspace  VariableName=Pe  SampleTime=1/60
  W3 : ToWorkspace  VariableName=DTH  SampleTime=1/60
  W4 : ToWorkspace  VariableName=Vt  SampleTime=1/60
  W5 : ToWorkspace  VariableName=PSS  SampleTime=1/60
  W6 : ToWorkspace  VariableName=EFD  SampleTime=1/60
  W7 : ToWorkspace  VariableName=t  SampleTime=1/60
  d_theta : Outport  VectorParamsAs1DForOutWhenUnconnected=off
  w : Outport  Port=2  VectorParamsAs1DForOutWhenUnconnected=off
  Pa : Outport  Port=3  VectorParamsAs1DForOutWhenUnconnected=off
  Vt : Outport  Port=4  VectorParamsAs1DForOutWhenUnconnected=off
  Stop : Outport  Port=5  VectorParamsAs1DForOutWhenUnconnected=off
  wires:
  Mux1/1 -> Sum3/1, W3/1, d_theta/1  "d_theta"
  Abs/1 -> MinMax/1
  Pref2/1 -> Relational Operator/2
  MinMax/1 -> Relational Operator/1
  [Pa1] -> Mux2/1
  Mux4/1 -> "Stability Signals Yellow=G1 mag=G2 cyan=G3 red=G4 "/1, W5/1  "pss"
  [pss1] -> Mux4/1
  [pss2] -> Mux4/2
  [pss4] -> Mux4/4
  [pss3] -> Mux4/3
  [EFD1] -> Mux6/1
  [EFD2] -> Mux6/2
  [EFD4] -> Mux6/4
  [EFD3] -> Mux6/3
  Mux6/1 -> Field Voltage Yellow=G1 mag=G2 cyan=G3 red=G4 green=CS1/1, W6/1
  Mux8/1 -> w/1, W/1  "w"
  Relational Operator/1 -> Stop/1
  Mux2/1 -> Pa/1, W1/1  "Pa"
  [theta1] -> Gain/1
  Gain/1 -> Scope/1, Mux1/1
  [theta2] -> Gain1/1
  [theta3] -> Gain2/1
  [theta4] -> Gain3/1
  Gain1/1 -> Mux1/2
  Gain2/1 -> Mux1/3
  [Pa2] -> Mux2/2
  [Pa3] -> Mux2/3
  [Pa4] -> Mux2/4
  [Vt1] -> Mux3/1
  [Vt2] -> Mux3/2
  [Vt3] -> Mux3/3
  [Vt4] -> Mux3/4
  Mux3/1 -> Vt/1, W4/1  "Vt"
  [Pe1] -> Mux5/1
  [Pe2] -> Mux5/2
  [Pe3] -> Mux5/3
  [Pe4] -> Mux5/4
  Mux5/1 -> "Electrical Power Yellow=M1 mag=M2 cyan=M3 red=M4 "/1, W2/1  "Pe"
  [w1] -> Mux8/1
  [w2] -> Mux8/2
  [w3] -> Mux8/3
  [w4] -> Mux8/4
  Clock/1 -> W7/1
  Gain3/1 -> Sum3/2, Mux1/4
  Sum3/1 -> Abs/1

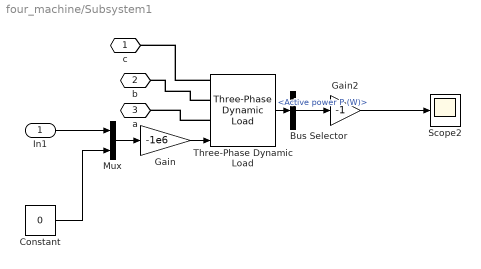
== system four_machine/Subsystem1 ==
  In1 : Inport
  Bus Selector : BusSelector  OutputSignals=Active power P (W)
  Constant : Constant  Value=0
  Gain : Gain  Gain=-1e6
  Gain2 : Gain  Gain=-1
  Mux : Mux  Inputs=2
  Scope2 : Scope
  Three-Phase Dynamic Load : powerlib/Elements/Three-Phase Dynamic Load  NominalVoltage=[ 230e3 60 ]  ActiveReactivePowers=[1e-06 1e-06]  PositiveSequence=[0.965022 13.4497]  ExternalControl=on  NpNq=[1.3 2]  TimeConstants="[0  0  0  0]"  MinimumVoltage=0.7  Tfilter=1e-4  LoadFlowParameters=[4,0,0,0,0]
      settings: SourceProductBaseCode=PS
  c : PMIOPort  Side=Left
  b : PMIOPort  Port=2  Side=Left
  a : PMIOPort  Port=3  Side=Left
  wires:
  Bus Selector/1 -> Gain2/1  "<Active power P (W)>"
  Three-Phase Dynamic Load/1 -> Bus Selector/1
  Mux/1 -> Gain/1
  Constant/1 -> Mux/2
  Gain/1 -> Three-Phase Dynamic Load/1
  In1/1 -> Mux/1
  Gain2/1 -> Scope2/1
  connections:
  Three-Phase Dynamic Load/LConn2 -- b/RConn1
  Three-Phase Dynamic Load/LConn3 -- c/RConn1
  Three-Phase Dynamic Load/LConn1 -- a/RConn1

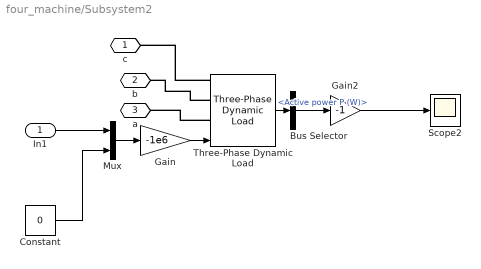
== system four_machine/Subsystem2 ==
  In1 : Inport
  Bus Selector : BusSelector  OutputSignals=Active power P (W)
  Constant : Constant  Value=0
  Gain : Gain  Gain=-1e6
  Gain2 : Gain  Gain=-1
  Mux : Mux  Inputs=2
  Scope2 : Scope
  Three-Phase Dynamic Load : powerlib/Elements/Three-Phase Dynamic Load  NominalVoltage=[ 230e3 60 ]  ActiveReactivePowers=[1e-06 1e-06]  PositiveSequence=[0.97603 -23.7392]  ExternalControl=on  NpNq=[1.3 2]  TimeConstants="[0  0  0  0]"  MinimumVoltage=0.7  Tfilter=1e-4  LoadFlowParameters=[4,0,0,0,0]
      settings: SourceProductBaseCode=PS
  c : PMIOPort  Side=Left
  b : PMIOPort  Port=2  Side=Left
  a : PMIOPort  Port=3  Side=Left
  wires:
  Bus Selector/1 -> Gain2/1  "<Active power P (W)>"
  Three-Phase Dynamic Load/1 -> Bus Selector/1
  Mux/1 -> Gain/1
  Constant/1 -> Mux/2
  Gain/1 -> Three-Phase Dynamic Load/1
  In1/1 -> Mux/1
  Gain2/1 -> Scope2/1
  connections:
  Three-Phase Dynamic Load/LConn2 -- b/RConn1
  Three-Phase Dynamic Load/LConn3 -- c/RConn1
  Three-Phase Dynamic Load/LConn1 -- a/RConn1

== system four_machine/Subsystem3 ==
  input : Inport
  Step2 : Step  Time=1e-9  Before=1  After=0  SampleTime=0  ZeroCross=off
  Subsystem : Subsystem  AncestorBlock="Nordic32_Lib/PSS  Nordic32/Subsystem"
  Subtract : Sum  Inputs=+-
  output : Outport  VectorParamsAs1DForOutWhenUnconnected=off
  wires:
  Step2/1 -> Subsystem/Enable
  Subsystem/1(y) -> Subtract/2  "Pe0"
  input/1 -> Subtract/1, Subsystem/1(u)
  Subtract/1 -> output/1

== system four_machine/Subsystem4 ==
  input : Inport
  Step2 : Step  Time=1e-9  Before=1  After=0  SampleTime=0  ZeroCross=off
  Subsystem : Subsystem  AncestorBlock="Nordic32_Lib/PSS  Nordic32/Subsystem"
  Subtract : Sum  Inputs=+-
  output : Outport  VectorParamsAs1DForOutWhenUnconnected=off
  wires:
  Step2/1 -> Subsystem/Enable
  Subsystem/1(y) -> Subtract/2  "Pe0"
  input/1 -> Subtract/1, Subsystem/1(u)
  Subtract/1 -> output/1

== system four_machine/Subsystem5 ==
  input : Inport
  Step2 : Step  Time=1e-9  Before=1  After=0  SampleTime=0  ZeroCross=off
  Subsystem : Subsystem  AncestorBlock="Nordic32_Lib/PSS  Nordic32/Subsystem"
  Subtract : Sum  Inputs=+-
  output : Outport  VectorParamsAs1DForOutWhenUnconnected=off
  wires:
  Step2/1 -> Subsystem/Enable
  Subsystem/1(y) -> Subtract/2  "Pe0"
  input/1 -> Subtract/1, Subsystem/1(u)
  Subtract/1 -> output/1

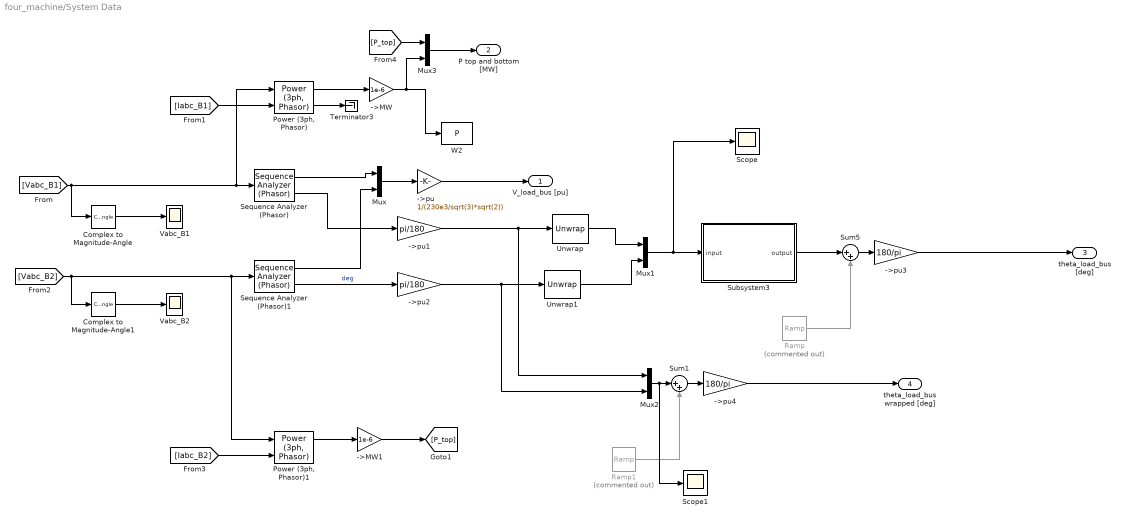
== system four_machine/System Data ==
  ->MW : Gain  Gain=1e-6  SaturateOnIntegerOverflow=on  OutDataTypeStr=Inherit: Same as input  ParamDataTypeStr=Inherit: Same as input
  ->MW1 : Gain  Gain=1e-6  SaturateOnIntegerOverflow=on  OutDataTypeStr=Inherit: Same as input  ParamDataTypeStr=Inherit: Same as input
  ->pu : Gain  Gain=1/(230e3/sqrt(3)*sqrt(2))  SaturateOnIntegerOverflow=on  OutDataTypeStr=Inherit: Same as input  ParamDataTypeStr=Inherit: Same as input
  ->pu1 : Gain  Gain=pi/180  SaturateOnIntegerOverflow=on  OutDataTypeStr=Inherit: Same as input  ParamDataTypeStr=Inherit: Same as input
  ->pu2 : Gain  Gain=pi/180  SaturateOnIntegerOverflow=on  OutDataTypeStr=Inherit: Same as input  ParamDataTypeStr=Inherit: Same as input
  ->pu3 : Gain  Gain=180/pi  SaturateOnIntegerOverflow=on  OutDataTypeStr=Inherit: Same as input  ParamDataTypeStr=Inherit: Same as input
  ->pu4 : Gain  Gain=180/pi  SaturateOnIntegerOverflow=on  OutDataTypeStr=Inherit: Same as input  ParamDataTypeStr=Inherit: Same as input
  Complex to Magnitude-Angle : ComplexToMagnitudeAngle  Output=Magnitude
  Complex to Magnitude-Angle1 : ComplexToMagnitudeAngle  Output=Magnitude
  Mux{,1..3} (4 alike) : Mux  Inputs=2
  "Power (3ph, Phasor)" : powerlib_meascontrol/Measurements/Power (3ph, Phasor)
      settings: SourceProductBaseCode=PS
  "Power (3ph, Phasor)1" : powerlib_meascontrol/Measurements/Power (3ph, Phasor)
      settings: SourceProductBaseCode=PS
  Ramp : simulink/Sources/Ramp  Commented=on  slope=60*2*pi  start=0  InitialOutput=0
  Ramp1 : simulink/Sources/Ramp  Commented=on  slope=60*2*pi  start=0  InitialOutput=0
  Scope : Scope
  Scope1 : Scope
  Sequence Analyzer (Phasor) : powerlib_meascontrol/Measurements/Sequence Analyzer (Phasor)  seq=Positive
      settings: SourceProductBaseCode=PS
  Sequence Analyzer (Phasor)1 : powerlib_meascontrol/Measurements/Sequence Analyzer (Phasor)  seq=Positive
      settings: SourceProductBaseCode=PS
  Subsystem3 : Subsystem
  Sum1 : Sum  Inputs=|++
  Sum5 : Sum  Inputs=|++
  Terminator3 : Terminator
  Unwrap : dspsigops/Unwrap  tol=pi  InputProcessing=Columns as channels (frame based)  running=off
  Unwrap1 : dspsigops/Unwrap  tol=pi  InputProcessing=Columns as channels (frame based)  running=off
  Vabc_B1 : Scope
  Vabc_B2 : Scope
  W2 : ToWorkspace  VariableName=P  SampleTime=1/60
  V_load_bus [pu] : Outport  VectorParamsAs1DForOutWhenUnconnected=off
  P top and bottom [MW] : Outport  Port=2  VectorParamsAs1DForOutWhenUnconnected=off
  theta_load_bus [deg] : Outport  Port=3  VectorParamsAs1DForOutWhenUnconnected=off
  theta_load_bus wrapped [deg] : Outport  Port=4  VectorParamsAs1DForOutWhenUnconnected=off
  wires:
  [Vabc_B1] -> Sequence Analyzer (Phasor)/1, "Power (3ph, Phasor)"/1, Complex to Magnitude-Angle/1
  [Iabc_B2] -> "Power (3ph, Phasor)1"/2
  Sequence Analyzer (Phasor)1/1 -> Mux/2
  [Iabc_B1] -> "Power (3ph, Phasor)"/2
  ->pu/1 -> V_load_bus [pu]/1
  Sequence Analyzer (Phasor)/1 -> Mux/1
  Mux/1 -> ->pu/1
  ->MW/1 -> Mux3/2, W2/1
  Complex to Magnitude-Angle/1 -> Vabc_B1/1
  Complex to Magnitude-Angle1/1 -> Vabc_B2/1
  "Power (3ph, Phasor)"/1 -> ->MW/1
  "Power (3ph, Phasor)"/2 -> Terminator3/1
  [Vabc_B2] -> "Power (3ph, Phasor)1"/1, Sequence Analyzer (Phasor)1/1, Complex to Magnitude-Angle1/1
  Sequence Analyzer (Phasor)1/2 -> ->pu2/1  "deg"
  Sequence Analyzer (Phasor)/2 -> ->pu1/1
  Mux1/1 -> Scope/1, Subsystem3/1(input)
  Ramp/1 -> Sum5/2
  Sum5/1 -> ->pu3/1
  ->pu1/1 -> Mux2/1, Unwrap/1
  Unwrap/1 -> Mux1/1
  Unwrap1/1 -> Mux1/2
  ->pu3/1 -> theta_load_bus [deg]/1
  ->pu2/1 -> Mux2/2, Unwrap1/1
  Sum1/1 -> ->pu4/1
  Ramp1/1 -> Sum1/2
  Mux2/1 -> Scope1/1, Sum1/1
  ->pu4/1 -> theta_load_bus wrapped [deg]/1
  Subsystem3/1(output) -> Sum5/1
  "Power (3ph, Phasor)1"/1 -> ->MW1/1
  ->MW1/1 -> [P_top]
  [P_top] -> Mux3/1
  Mux3/1 -> P top and bottom [MW]/1

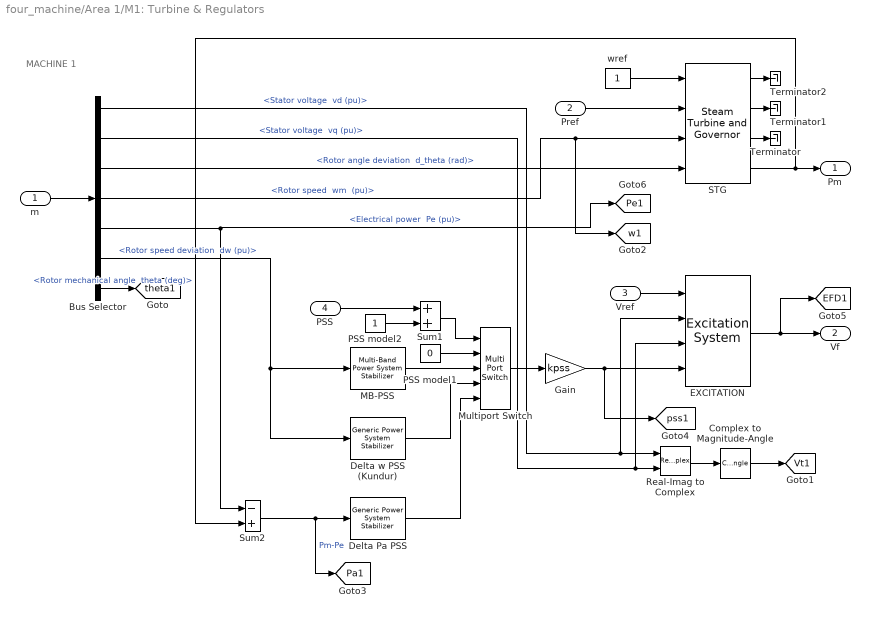
== system four_machine/Area 1/M1: Turbine & Regulators ==
  note: MACHINE 1
  m : Inport
  Pref : Inport  Port=2
  Vref : Inport  Port=3
  PSS : Inport  Port=4
  Bus Selector : BusSelector  OutputSignals="dq0 components.Stator voltage  vd (pu),dq0 components.Stator voltage  vq (pu),Mechanical.Rotor angle deviation  d_theta (rad),Mechanical.Rotor speed  wm  (pu),Mechanical.Electrical power  Pe (pu),Mechanical.Rotor speed deviation  dw (pu),Mechanical.Rotor mechanical angle  theta (deg)"
  Complex to Magnitude-Angle : ComplexToMagnitudeAngle  Output=Magnitude
  "Delta Pa PSS " : powerlib/Machines/Generic Power System Stabilizer  Tsensor=15e-3  K=2.5*1.25  Twashout=1  Tleadlag1=[60e-3 1]  Tleadlag2=[0 0]  VSlimits=[-0.15 0.15]  Vinit=0  Plot_On=off  MagdB_On=off  FreqRange=logspace(-2,2,500)
      settings: SourceProductBaseCode=PS
  "Delta w PSS (Kundur) " : powerlib/Machines/Generic Power System Stabilizer  Tsensor=15e-3  K=30  Twashout=10  Tleadlag1=[50e-3 20e-3]  Tleadlag2=[3 5.4]  VSlimits=[-0.15 0.15]  Vinit=0  Plot_On=off  MagdB_On=off  FreqRange=logspace(-2,2,500)
      settings: SourceProductBaseCode=PS
  EXCITATION : sps_avr/Excitation System  tr=20e-3  reg=[ 200, 0.001 ]  exc=[ 1, 0 ]  tgr=[ 0, 0 ]  damp=[ 0, 0 ]  sat=[ 0, 0 ]  lim=[ 0 , 12.3, 0 ]  v0=[1 1.8845]
      settings: SourceProductBaseCode=PS
  Gain : Gain  Gain=kpss
  "MB-PSS " : powerlib/Machines/Multi-Band Power System Stabilizer  OperationMode=Simplified settings  Kg=1.0  GL=[0.2 30]  GI=[1.25 40]  GH=[12.0 160]  GLd=[66 66 9.4]  TcLF=[1.667 2 0 0 0 0 2 2.4 0 0 0 0 1 1]  GId=[66 66 47.6]  TcIF=[1 1 0.25 0.3 0 0 1 1 0.3 0.36 0 0 0 0]  GHd=[66 66 233]  TcHF="[0.01 0.012 0 0 0 0  0.012 0.0144 0 0 0 0 1 1]"  LIM=[.075 .15 .15 .15]  Plot_On=off  MagdB_On=off  FreqRange=logspace(-2,2,500)
      settings: SourceProductBaseCode=PS
  Multiport Switch : MultiPortSwitch  Inputs=4  InputSameDT=on
  PSS model1 : Constant  Value=0
  PSS model2 : Constant
  Real-Imag to Complex : RealImagToComplex
  STG : powerlib/Machines/Steam Turbine and Governor  gentype=Tandem-compound (single mass)  reg1="[ 1  0.05    0 ]"  reg2="[ 0.001  0.15 ]"  reg3="[ -0.1  0.1  0  4.496 ]"  N=3600  turb1="[ 0  10   3.3   0.5   ]"  turb2="[   0   0.36    0.36   0.28   ]"  HA="[ 0.046  1.430  1.465   0.192 ]"  KA="[ 90.44  53.88  64.59   62.94  ]"  DA="[ 0.0115  0.3575  0.3663   0.0137  ]"  ini1=0.77934  ini2=[0.779316,-31.4247]
      settings: SourceProductBaseCode=PS
  Sum1 : Sum  InputSameDT=on  SaturateOnIntegerOverflow=on  OutDataTypeStr=Inherit: Same as first input
  Sum2 : Sum  Inputs=-+  InputSameDT=on  SaturateOnIntegerOverflow=on  OutDataTypeStr=Inherit: Same as first input
  Terminator : Terminator
  Terminator1 : Terminator
  Terminator2 : Terminator
  wref : Constant
  Pm : Outport  InitialOutput=0  VectorParamsAs1DForOutWhenUnconnected=off
  Vf : Outport  Port=2  InitialOutput=0  VectorParamsAs1DForOutWhenUnconnected=off
  tag scope: EFD1=global, Pa1=global, Pe1=global, Vt1=global, pss1=global, theta1=global, w1=global
  wires:
  Bus Selector/1 -> Real-Imag to Complex/1, EXCITATION/2  "<Stator voltage  vd (pu)>"
  Bus Selector/2 -> Real-Imag to Complex/2, EXCITATION/3  "<Stator voltage  vq (pu)>"
  wref/1 -> STG/1
  Pref/1 -> STG/2
  m/1 -> Bus Selector/1
  Vref/1 -> EXCITATION/1
  Real-Imag to Complex/1 -> Complex to Magnitude-Angle/1
  EXCITATION/1 -> Vf/1, [EFD1]
  Complex to Magnitude-Angle/1 -> [Vt1]
  Bus Selector/7 -> [theta1]  "<Rotor mechanical angle  theta (deg)>"
  Multiport Switch/1 -> Gain/1
  PSS model1/1 -> Multiport Switch/2
  "MB-PSS "/1 -> Multiport Switch/3
  "Delta w PSS (Kundur) "/1 -> Multiport Switch/4
  "Delta Pa PSS "/1 -> Multiport Switch/5
  PSS model2/1 -> Sum1/2
  Sum1/1 -> Multiport Switch/1
  PSS/1 -> Sum1/1
  Bus Selector/4 -> [w1], STG/3  "<Rotor speed  wm  (pu)>"
  Bus Selector/5 -> [Pe1], Sum2/1  "<Electrical power  Pe (pu)>"
  Bus Selector/6 -> "Delta w PSS (Kundur) "/1, "MB-PSS "/1  "<Rotor speed deviation  dw (pu)>"
  Sum2/1 -> [Pa1], "Delta Pa PSS "/1  "Pm-Pe"
  STG/3 -> Terminator/1
  STG/4 -> Pm/1, Sum2/2
  STG/2 -> Terminator1/1
  STG/1 -> Terminator2/1
  Bus Selector/3 -> STG/4  "<Rotor angle deviation  d_theta (rad)>"
  Gain/1 -> EXCITATION/4, [pss1]
